simulink model "ModelFor12Vbattery"  (R2015a)
settings: Solver=ode45  StartTime=0.0  StopTime=10.0  RelTol=1e-3
undefined symbols (not defined in the file or in its folder): Acid, Lead
libraries: powerlib x10, simulink x2, powerlib_meascontrol x2, electricdrivelib x1, nesl_utility x1
settings Model: Creator=Tushar  LastModifiedBy=Tushar

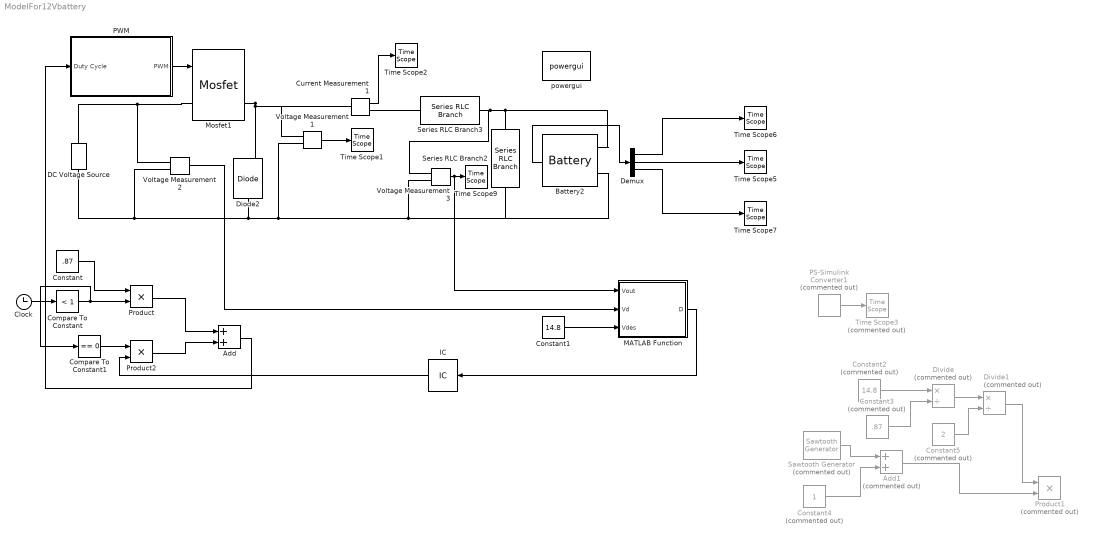
== system ModelFor12Vbattery ==
  Add : Sum
  Add1 : Sum  Commented=on
  Battery2 : electricdrivelib/Extra Sources/Battery  BatType=Lead-Acid  ShowDetailedParameters=off  NomV=12  NomQ=18  SOC=0  PresetModel=on  MaxQ=18.75  FullV=13.0658  Dis_rate=3.6  R=0.0066667  Normal_OP=5.585  expZone="[12.2171         0.06]"  current=[6.5 13 32.5]  Units=Time  Batt_Tr=10e-6
  Clock : Clock
  Compare To Constant : simulink/Logic and Bit Operations/Compare To Constant  relop=<  const=1  OutDataTypeStr=boolean
  Compare To Constant1 : simulink/Logic and Bit Operations/Compare To Constant  relop===  const=0  OutDataTypeStr=boolean
  Constant : Constant  Value=.87
  Constant1 : Constant  Value=14.8
  Constant2 : Constant  Commented=on  Value=14.8
  Constant3 : Constant  Commented=on  Value=.87
  Constant4 : Constant  Commented=on
  Constant5 : Constant  Commented=on  Value=2
  Current Measurement1 : powerlib/Measurements/Current Measurement  PhasorSimulation=off  OutputType=Complex  PSBequivalent=0
  DC Voltage Source : powerlib/Electrical Sources/DC Voltage Source  Amplitude=25  Measurements=Voltage
  Demux : Demux  Outputs=3
  Diode2 : powerlib/Power Electronics/Diode  Ron=0.00001  Lon=0  Vf=0  IC=0  UseSnubber=off  Rs=500  Cs=250e-9  Measurements=on
  Divide : Product  Commented=on  Inputs=*/
  Divide1 : Product  Commented=on  Inputs=*/
  IC : InitialCondition
  MATLAB Function : MATLAB Function  TreatAsAtomicUnit=on
  Mosfet1 : powerlib/Power Electronics/Mosfet  Ron=0.0001  Lon=0  Rd=0.001  Vfd=0  IC=0  Rs=42  Cs=600e-12  Measurements=on
  PS-Simulink Converter1 : nesl_utility/PS-Simulink Converter  Commented=on  PhysicalDomain=network_engine_domain  SubClassName=ps_output  LeftPortType=input  RightPortType=output  PseudoPeriodic=off  Frequencies=[]  Unit=V  AffineConversion=off
  PWM : Subsystem
  Product : Product
  Product1 : Product  Commented=on
  Product2 : Product
  Sawtooth Generator : powerlib_meascontrol/Pulse & Signal Generators/Sawtooth Generator  Commented=on  Freq=40000  Phase=0  Ts=0
  Series RLC Branch2 : powerlib/Elements/Series RLC Branch  LConnTagsString=__new0  RConnTagsString=__new0  BranchType=RC  Resistance=.0015  Inductance=1e-3  SetiL0=off  InitialCurrent=0  Capacitance=100e-6  Setx0=on  InitialVoltage=0  Measurements=Branch voltage
  Series RLC Branch3 : powerlib/Elements/Series RLC Branch  LConnTagsString=__new0  RConnTagsString=__new0  BranchType=RL  Resistance=1.4e-3  Inductance=420e-6  SetiL0=off  InitialCurrent=0  Capacitance=1e-6  Setx0=off  InitialVoltage=0  Measurements=None
  Time Scope{1..2,5..7,9} (6 alike) : TimeScope  DefaultConfigurationName=spbscopes.TimeScopeBlockCfg
  Time Scope3 : TimeScope  Commented=on  DefaultConfigurationName=spbscopes.TimeScopeBlockCfg
  Voltage Measurement1 : powerlib/Measurements/Voltage Measurement  PhasorSimulation=off  OutputType=Complex  PSBequivalent=0
  Voltage Measurement2 : powerlib/Measurements/Voltage Measurement  PhasorSimulation=off  OutputType=Complex  PSBequivalent=0
  Voltage Measurement3 : powerlib/Measurements/Voltage Measurement  PhasorSimulation=off  OutputType=Complex  PSBequivalent=0
  powergui : powerlib/powergui  Priority=1  SimulationMode=Discrete  SolverType=Tustin/Backward Euler (TBE)  SampleTime=10e-7  frequency=60  SPID=off  DisableSnubberDevices=off  DisableRonSwitches=off  DisableVfSwitches=off  SwTol=0  DisplayEquations=off  Interpol=off  methode=off  Ts=100  FunctionMessages=off  echomessages=off  HookPort=off  EnableUseOfTLC=off  x0status=blocks  frequencyindice=0  Pbase=100e6  ErrMax=1e-4  Iterations=50  UnitsV=kV  UnitsW=MW  buscounter=0  RestoreLinks=warning  ResistiveCurrentMeasurement=off  Frange=[0:2:500]  Ylog=off  Xlog=on  ShowGrid=off  save=off  variable=ZData  structure=0  ZoomFFT=off  StartTime=0.0  cycles=1  DisplayStyle=1  fundamental=60  FreqAxis=off  MaxFrequency=1000  frequencyindicesteady=1  RmsSteady=1  display=off
  wires:
  PWM/1(PWM) -> Mosfet1/1
  Current Measurement1/1 -> Time Scope2/1
  Voltage Measurement3/1 -> MATLAB Function/1(Vout), Time Scope9/1
  Voltage Measurement1/1 -> Time Scope1/1
  Sawtooth Generator/1 -> Add1/1
  Constant4/1 -> Add1/2
  Add1/1 -> Product1/2
  Constant2/1 -> Divide/1
  Constant3/1 -> Divide/2
  Divide/1 -> Divide1/1
  Constant5/1 -> Divide1/2
  Divide1/1 -> Product1/1
  PS-Simulink Converter1/1 -> Time Scope3/1
  Battery2/1 -> Demux/1
  Demux/1 -> Time Scope6/1
  Demux/2 -> Time Scope5/1
  Demux/3 -> Time Scope7/1
  Voltage Measurement2/1 -> MATLAB Function/2(Vd)
  Constant1/1 -> MATLAB Function/3(Vdes)
  Clock/1 -> Compare To Constant/1
  Constant/1 -> Product/1
  Compare To Constant/1 -> Compare To Constant1/1, Product/2
  Compare To Constant1/1 -> Product2/1
  Product/1 -> Add/1
  Product2/1 -> Add/2
  Add/1 -> PWM/1("Duty Cycle ")
  IC/1 -> Product2/2
  MATLAB Function/1(D) -> IC/1
  connections:
  Voltage Measurement3/LConn1 -- Series RLC Branch3/RConn1 -- Battery2/LConn1 -- Series RLC Branch2/LConn1
  Mosfet1/RConn1 -- Diode2/RConn1 -- Current Measurement1/LConn1 -- Voltage Measurement1/LConn1
  Diode2/LConn1 -- Voltage Measurement1/LConn2 -- Voltage Measurement3/LConn2 -- Series RLC Branch2/RConn1 -- Battery2/LConn2 -- Voltage Measurement2/LConn2 -- DC Voltage Source/LConn1
  DC Voltage Source/RConn1 -- Mosfet1/LConn1 -- Voltage Measurement2/LConn1
  Current Measurement1/RConn1 -- Series RLC Branch3/LConn1

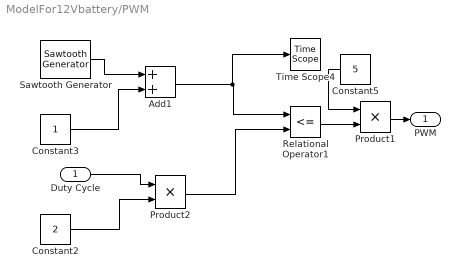
== system ModelFor12Vbattery/PWM ==
  "Duty Cycle " : Inport
  Add1 : Sum
  Constant2 : Constant  Value=2
  Constant3 : Constant
  Constant5 : Constant  Value=5
  Product1 : Product
  Product2 : Product
  Relational Operator1 : RelationalOperator  Operator=<=  OutDataTypeStr=boolean
  Sawtooth Generator : powerlib_meascontrol/Pulse & Signal Generators/Sawtooth Generator  Freq=40000  Phase=0  Ts=0
  Time Scope4 : TimeScope  DefaultConfigurationName=spbscopes.TimeScopeBlockCfg
  PWM : Outport
  wires:
  Relational Operator1/1 -> Product1/2
  Product2/1 -> Relational Operator1/2
  Sawtooth Generator/1 -> Add1/1
  Constant5/1 -> Product1/1
  Constant3/1 -> Add1/2
  Add1/1 -> Time Scope4/1, Relational Operator1/1
  Product1/1 -> PWM/1
  "Duty Cycle "/1 -> Product2/1
  Constant2/1 -> Product2/2

== matlab function ModelFor12Vbattery/MATLAB Function ==
  data: Vout input; D output; Vd input; Vdes input
function D = fcn(Vout,Vd,Vdes)
Dgiven=Vdes/Vd;
Dfound=Vout/Vd;
%#codegen
Derror=(Dgiven-Dfound)/Dgiven;
D=Dgiven/(1-Derror);
